simulink model "kalmnsce"  (Simulink 6.0)
settings: Solver=FixedStepDiscrete  SolverMode=SingleTasking  StartTime=0.0  StopTime=999999  RelTol=1e-3  AbsTol=1e-6
libraries: simulink x3, dsparch4 x2, dspindex x1, dspadpt3 x1, dspmtrx3 x1
Description:
  | Nonstationary channel estimation using a Kalman tracking filter
settings Model: CovMetricSettings=d  Creator=don  LastModifiedBy=navan  ExtModeTrigMode=oneshot  ExtModeArmWhenConnect=off
settings DataIOCC: LimitDataPoints=off  SaveOutput=off  SaveTime=off  SignalLoggingName=sigsOut
settings OptimizationCC: BlockReduction=off  BooleanDataType=off  MultiInstanced=off  RollThreshold=2
settings FormatCC: IgnoreBidirectionalLines=off
settings DebuggingCC: IntegerOverflowMsg=none
settings HardwareCC: TargetUnknown=on
settings CodeAppCC: FileBanners=off  CustomSymbols=off
settings GRTTargetCC: TargetFcnLib=iso_c_tmw.mat  IsERTTarget=off

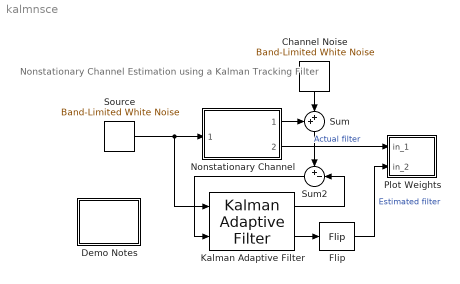
== system kalmnsce ==
  note: Nonstationary Channel Estimation
      | using a Kalman Tracking Filter
  Channel Noise : simulink/Sources/Band-Limited White Noise  Orientation=down  Cov=.3  Ts=1  seed=12345
  Demo Notes : Subsystem
      mask Display: disp('Info')
  Flip : dspindex/Flip  dim=Columns
  Kalman Adaptive Filter : dspadpt3/Kalman Adaptive Filter  Ntaps=5  Jmin=0.3  q=0.1  ic0=0  K0=0.5  Adapt=off  RstPort=None
  Nonstationary Channel : Subsystem  mask{N=5, a=0.96, Ts=1}
      mask prompts: N "Filter Order:"; a "Nonstationarity Parameter (0 to 1):"; Ts "Sample Time:"
      mask help: Nonstationary Nth Order Noisy Channel
      mask Help: Implementation of a nonstationary filter.  Nonstationarity parameter controls the filter tap nonstationarity, and may take values in the range 0 <= a < 1.  The first system output is the actual filter taps over time, and the second output is a vector of instantaneous tap weight estimates ("unknowns")
      mask Display: disp('Nonstationary\nSystem')
  Plot Weights : Subsystem
      mask Display: disp('Plot\nWeights')
  Source : simulink/Sources/Band-Limited White Noise  Cov=[0.1]  Ts=1  seed=[23341]
  Sum : Sum  Orientation=down  Inputs=++|  SaturateOnIntegerOverflow=on  InputSameDT=on
  Sum2 : Sum  Orientation=left  Inputs=+-|  SaturateOnIntegerOverflow=on  InputSameDT=on
  wires:
  Channel Noise/1 -> Sum/2
  Nonstationary Channel/1(Filter Output) -> Sum/1
  Source/1 -> Kalman Adaptive Filter/1, Nonstationary Channel/1(Input Signal)
  Nonstationary Channel/2(Tap Weights) -> Plot Weights/1(in_1)  "Actual filter"
  Kalman Adaptive Filter/1 -> Sum2/2
  Sum/1 -> Sum2/1
  Sum2/1 -> Kalman Adaptive Filter/2
  Kalman Adaptive Filter/2 -> Flip/1
  Flip/1 -> Plot Weights/2(in_2)  "Estimated filter"

== system kalmnsce/Demo Notes ==
  note: This demonstrates the ability of a Kalman filter to track
      | the time-varying weights of a nonstationary 5th order
      | FIR filter.
      |
      |  When run, a plot is made of each tap weight over time,
      | with the "true" filter taps drawn in yellow, and the
      | estimates of those tap weights in magenta.  Each of
      | the 5 tap weights is plotted in a separate axis.
      |
      | For more information on Kalman filtering, see
      | S. Haykin, "Adaptive Filter Theory",
      | 3rd Ed., Prentice Hall, 1996.
  note: Nonstationary Channel Estimation
      | using a Kalman Tracking Filter

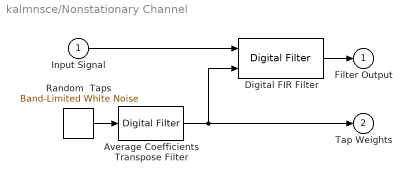
== system kalmnsce/Nonstationary Channel ==
  Input Signal : Inport
  Average Coefficients Transpose Filter : dsparch4/Digital Filter  TypePopup=IIR (all poles)  IIRFiltStruct=Direct form II transposed  AllPoleFiltStruct=Direct form transposed  FIRFiltStruct=Direct form  CoeffSource=Specify via dialog  NumCoeffs=[1 2]  DenCoeffs=[1 -a]  BiQuadCoeffs=[1 0.3 0.4 1 0.1 0.2]  LatticeCoeffs=[0.2 0.4]  denIgnore=on  FiltPerSampPopup=One filter per frame  IC=0  ICnum=0  ICden=0  roundingMode=Floor  overflowMode=off
  Digital FIR Filter : dsparch4/Digital Filter  TypePopup=FIR (all zeros)  IIRFiltStruct=Direct form II transposed  AllPoleFiltStruct=Direct form  FIRFiltStruct=Direct form transposed  CoeffSource=Input port(s)  NumCoeffs=[1 2]  DenCoeffs=[1 0.1]  BiQuadCoeffs=[1 0.3 0.4 1 0.1 0.2]  LatticeCoeffs=[0.2 0.4]  denIgnore=on  FiltPerSampPopup=One filter per sample  IC=0  ICnum=0  ICden=0  roundingMode=Floor  overflowMode=off
  Random  Taps : simulink/Sources/Band-Limited White Noise  Cov=ones(N,1)  Ts=Ts  seed=round(rand(N,1)*1000)
  Filter Output : Outport  InitialOutput=0
  Tap Weights : Outport  Port=2  InitialOutput=0
  wires:
  Input Signal/1 -> Digital FIR Filter/1
  Digital FIR Filter/1 -> Filter Output/1
  Random  Taps/1 -> Average Coefficients Transpose Filter/1
  Average Coefficients Transpose Filter/1 -> Tap Weights/1, Digital FIR Filter/2

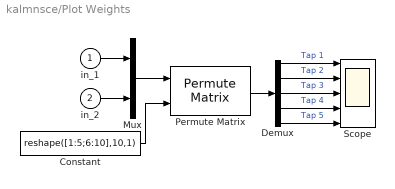
== system kalmnsce/Plot Weights ==
  in_1 : Inport
  in_2 : Inport  Port=2
  Constant : Constant  Value=reshape([1:5;6:10],10,1)
  Demux : Demux  Outputs=5
  Mux : Mux  Inputs=2
  Permute Matrix : dspmtrx3/Permute Matrix  mode=Rows  ZeroOneIdxMode=One-based  errmode=Clip Index  checkDims=off
  Scope : Scope  NumInputPorts=5
      settings: TimeRange=300  YMin=-10~-10~-10~-10~-10  YMax=10~10~10~10~10  DataFormat=Structure  SampleInput=on
  wires:
  Demux/5 -> Scope/5  "Tap 5"
  in_1/1 -> Mux/1
  in_2/1 -> Mux/2
  Mux/1 -> Permute Matrix/1
  Constant/1 -> Permute Matrix/2
  Permute Matrix/1 -> Demux/1
  Demux/1 -> Scope/1  "Tap 1"
  Demux/4 -> Scope/4  "Tap 4"
  Demux/3 -> Scope/3  "Tap 3"
  Demux/2 -> Scope/2  "Tap 2"
